simulink model "svpwm_model"  (R2024b)
settings: Solver=VariableStepAuto  StartTime=0.0  StopTime=10.0  RelTol=1e-3
undefined symbols (not defined in the file or in its folder): Ld, Lq, phi, pn
libraries: spsUniversalBridgeLib x1, spsPermanentMagnetSynchronousMachineLib x1, simulink x1, spsDCVoltageSourceLib x1, spsabctodq0Lib x1, spspowerguiLib x1

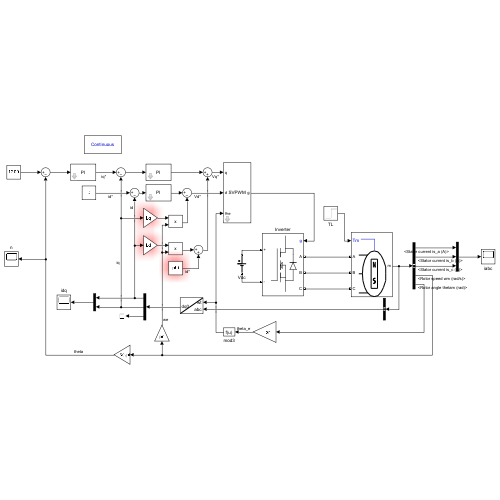
[thumbnail: Simulink's stored preview of the top-level diagram]
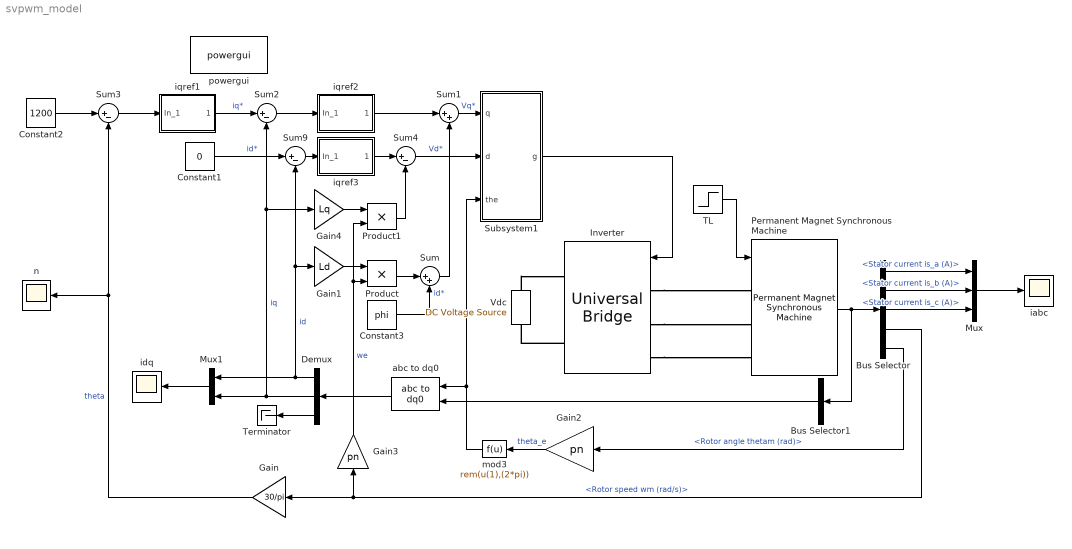
== system svpwm_model ==
  Bus Selector : BusSelector  OutputSignals=Stator current is_a (A),Stator current is_b (A),Stator current is_c (A),Rotor speed wm (rad/s),Rotor angle thetam (rad)
  Bus Selector1 : BusSelector  OutputSignals=Stator current is_a (A),Stator current is_b (A),Stator current is_c (A)  OutputAsBus=on
  Constant1 : Constant  Value=0
  Constant2 : Constant  Value=1200
  Constant3 : Constant  Value=phi
  Demux : Demux  Outputs=3
  Gain : Gain  Gain=30/pi
  Gain1 : Gain  Gain=Ld
  Gain2 : Gain  Gain=pn
  Gain3 : Gain  Gain=pn
  Gain4 : Gain  Gain=Lq
  Inverter : spsUniversalBridgeLib/Universal Bridge  Arms=3  SnubberResistance=1e5  SnubberCapacitance=inf  Device=MOSFET / Diodes  Ron=1e-3  Lon=0  ForwardVoltages="[  0  0  ]"  ForwardVoltage=0  GTOparameters=[ 10e-6 , 20e-6 ]  IGBTparameters=[ 1e-6 , 2e-6 ]  Measurements=None  Measurements_2=None  converterType=Rectifier
  Mux : Mux  Inputs=3
  Mux1 : Mux  Inputs=2
  Permanent Magnet Synchronous Machine : spsPermanentMagnetSynchronousMachineLib/Permanent Magnet Synchronous Machine  NbPhases=3  FluxDistribution=Sinusoidal  RotorType=Salient-pole  MechanicalLoad=Torque Tm  PresetModel="01:  0.8 Nm 300 Vdc 3000 RPM - 0.8 Nm"  ShowDetailedParameters=on  MeasurementBus=off  Resistance=18.7  Inductance=8.5e-3  dqInductances=[0.02547 0.02816]  La=0.000395  MachineConstant=Flux linkage established by magnets (V.s)  Flux=0.1716  VoltageCst=62.2496  TorqueCst=0.5148  Flat=120  Mechanical=[2.26e-05 1.349e-05 2 0]  PolePairs=2  InitialConditions=[0,0, 0,0]  InitialConditions5ph=[0 0 0 0 0 0]  RefAngle=Aligned with phase A axis (original Park)  IterativeDiscreteModel=Trapezoidal non iterative  TsBlock=-1  TsPowergui=0
  Product : Product
  Product1 : Product
  Subsystem1 : Subsystem  mask{Vdc=311}
  Sum : Sum  Inputs=|++
  Sum1 : Sum  Inputs=|++
  Sum{2..4,9} (4 alike) : Sum  Inputs=|+-
  TL : Step  Time=2  After=0.5  SampleTime=0
  Terminator : Terminator
  Vdc : spsDCVoltageSourceLib/DC Voltage Source  Amplitude=311  Measurements=None
  abc to dq0 : spsabctodq0Lib/abc to dq0  Alignment=Aligned with phase A axis
  iabc : Scope
  idq : Scope
  iqref1 : Subsystem  mask(PI Controller){I=20, P=0.15, sat=[-1, 1]}
      mask prompts: I "Integral"; P "Proportional:"; sat "Minimum and maximum outputs:"
      mask init:
      | min=sat(1);max=sat(2);
  iqref2 : Subsystem  mask(PI Controller){I=255, P=105, sat=[-311/2, 311/2]}
      mask prompts: I "Integral"; P "Proportional:"; sat "Minimum and maximum outputs:"
      mask init:
      | min=sat(1);max=sat(2);
  iqref3 : Subsystem  mask(PI Controller){I=255, P=105, sat=[-311/2,311/2]}
      mask prompts: I "Integral"; P "Proportional:"; sat "Minimum and maximum outputs:"
      mask init:
      | min=sat(1);max=sat(2);
  mod3 : Fcn  Expr=rem(u(1),(2*pi))
  n : Scope
  powergui : spspowerguiLib/powergui  Priority=1  SimulationMode=Continuous  SampleTime=10e-6  frequency=60  Iterations=50  frequencyindice=0  Pbase=100e6  ErrMax=1e-4  UnitsV=kV  UnitsW=MW  buscounter=0  FunctionMessages=off  echomessages=off  EnableUseOfTLC=off  CurrentSourceSwitches=off  DisableSnubberDevices=off  DisableRonSwitches=off  DisableVfSwitches=off  DisplayEquations=off  AutomaticDiscreteSolvers=off  SolverType=Tustin/Backward Euler (TBE)  Interpol=off  ExternalGateDelay=off  methode=off  Ts=100  x0status=blocks  SPID=on  SwTol=0  HookPort=off  NonlinearTolerance=1e-4  nMaxIteration=100  ContinueOnMaxIteration=off  RestoreLinks=warning  ResistiveCurrentMeasurement=off  Frange=[0:2:500]  Ylog=off  Xlog=on  ShowGrid=off  save=off  variable=ZData  structure=0  ZoomFFT=off  StartTime=0.0  cycles=1  DisplayStyle=1  fundamental=60  FreqAxis=off  MaxFrequency=1000  frequencyindicesteady=1  RmsSteady=1  display=off
  wires:
  Sum3/1 -> iqref1/1(In_1)
  Bus Selector/1 -> Mux/1  "<Stator current is_a (A)>"
  Mux/1 -> iabc/1
  abc to dq0/1 -> Demux/1
  Constant1/1 -> Sum9/1  "id*"
  Bus Selector/2 -> Mux/2  "<Stator current is_b (A)>"
  Gain/1 -> Sum3/2, n/1  "theta"
  iqref1/1(Out_1) -> Sum2/1  "iq*"
  mod3/1 -> Subsystem1/3(the), abc to dq0/2
  Bus Selector/4 -> Gain3/1, Gain/1  "<Rotor speed wm (rad/s)>"
  Demux/2 -> Sum2/2, Gain4/1, Mux1/2  "iq"
  Demux/3 -> Terminator/1
  Mux1/1 -> idq/1
  Subsystem1/1(g) -> Inverter/1
  Bus Selector/5 -> Gain2/1  "<Rotor angle thetam (rad)>"
  Sum9/1 -> iqref3/1(In_1)
  Sum2/1 -> iqref2/1(In_1)
  Bus Selector/3 -> Mux/3  "<Stator current is_c (A)>"
  Gain2/1 -> mod3/1  "theta_e"
  Bus Selector1/1 -> abc to dq0/1
  Constant2/1 -> Sum3/1
  TL/1 -> Permanent Magnet Synchronous Machine/1
  Permanent Magnet Synchronous Machine/1 -> Bus Selector1/1, Bus Selector/1
  Demux/1 -> Sum9/2, Gain1/1, Mux1/1  "id"
  iqref2/1(Out_1) -> Sum1/1
  Sum1/1 -> Subsystem1/1(q)  "Vq*"
  Gain3/1 -> Product1/2, Product/2  "we"
  Gain1/1 -> Product/1
  Product/1 -> Sum/1
  Constant3/1 -> Sum/2  "id*"
  Sum/1 -> Sum1/2
  iqref3/1(Out_1) -> Sum4/1
  Gain4/1 -> Product1/1
  Product1/1 -> Sum4/2
  Sum4/1 -> Subsystem1/2(d)  "Vd*"
  connections:
  Inverter/LConn2 -- Permanent Magnet Synchronous Machine/LConn2
  Inverter/LConn1 -- Permanent Magnet Synchronous Machine/LConn1
  Vdc/RConn1 -- Inverter/RConn1
  Inverter/LConn3 -- Permanent Magnet Synchronous Machine/LConn3
  Inverter/RConn2 -- Vdc/LConn1

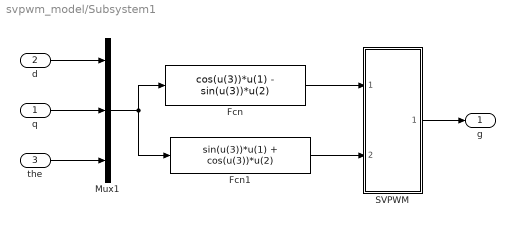
== system svpwm_model/Subsystem1 ==
  q : Inport
  d : Inport  Port=2
  the : Inport  Port=3
  Fcn : Fcn  Expr=cos(u(3))*u(1) - sin(u(3))*u(2)
  Fcn1 : Fcn  Expr=sin(u(3))*u(1) + cos(u(3))*u(2)
  Mux1 : Mux  Inputs=3
  SVPWM : Subsystem  Tag=SVPWM  mask{F=10, Vdc=311}
      mask prompts: F "Chopping　Frequency(KHz)"; Vdc "DC Voltage(V)"
  g : Outport
  wires:
  q/1 -> Mux1/2
  Fcn/1 -> SVPWM/1(Ualfa)
  d/1 -> Mux1/1
  Fcn1/1 -> SVPWM/2(Ubeta)
  SVPWM/1(pulse) -> g/1
  Mux1/1 -> Fcn/1, Fcn1/1
  the/1 -> Mux1/3

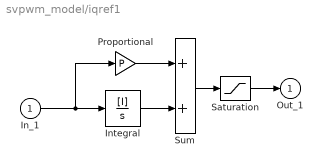
== system svpwm_model/iqref1 ==
  In_1 : Inport
  Integral : TransferFcn  Numerator=[I]  Denominator=[1 0]
  Proportional : Gain  Gain=P  SaturateOnIntegerOverflow=on  OutDataTypeStr=Inherit: Same as input  ParamDataTypeStr=Inherit: Same as input
  Saturation : Saturate  UpperLimit=max  LowerLimit=min
  Sum : Sum  InputSameDT=on  SaturateOnIntegerOverflow=on  OutDataTypeStr=Inherit: Same as first input
  Out_1 : Outport  InitialOutput=0  VectorParamsAs1DForOutWhenUnconnected=off
  wires:
  Saturation/1 -> Out_1/1
  Sum/1 -> Saturation/1
  Proportional/1 -> Sum/1
  In_1/1 -> Proportional/1, Integral/1
  Integral/1 -> Sum/2

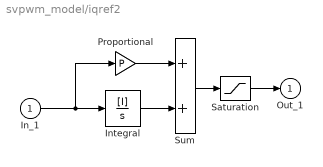
== system svpwm_model/iqref2 ==
  In_1 : Inport
  Integral : TransferFcn  Numerator=[I]  Denominator=[1 0]
  Proportional : Gain  Gain=P  SaturateOnIntegerOverflow=on  OutDataTypeStr=Inherit: Same as input  ParamDataTypeStr=Inherit: Same as input
  Saturation : Saturate  UpperLimit=max  LowerLimit=min
  Sum : Sum  InputSameDT=on  SaturateOnIntegerOverflow=on  OutDataTypeStr=Inherit: Same as first input
  Out_1 : Outport  InitialOutput=0  VectorParamsAs1DForOutWhenUnconnected=off
  wires:
  Saturation/1 -> Out_1/1
  Sum/1 -> Saturation/1
  Proportional/1 -> Sum/1
  In_1/1 -> Proportional/1, Integral/1
  Integral/1 -> Sum/2

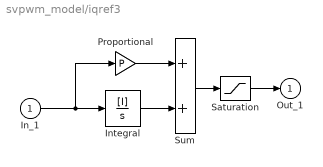
== system svpwm_model/iqref3 ==
  In_1 : Inport
  Integral : TransferFcn  Numerator=[I]  Denominator=[1 0]
  Proportional : Gain  Gain=P  SaturateOnIntegerOverflow=on  OutDataTypeStr=Inherit: Same as input  ParamDataTypeStr=Inherit: Same as input
  Saturation : Saturate  UpperLimit=max  LowerLimit=min
  Sum : Sum  InputSameDT=on  SaturateOnIntegerOverflow=on  OutDataTypeStr=Inherit: Same as first input
  Out_1 : Outport  InitialOutput=0  VectorParamsAs1DForOutWhenUnconnected=off
  wires:
  Saturation/1 -> Out_1/1
  Sum/1 -> Saturation/1
  Proportional/1 -> Sum/1
  In_1/1 -> Proportional/1, Integral/1
  Integral/1 -> Sum/2

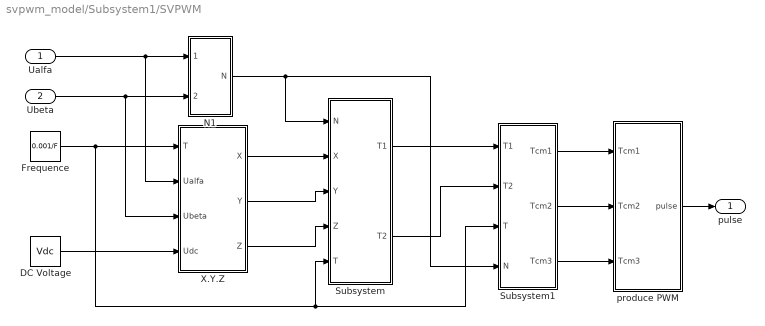
== system svpwm_model/Subsystem1/SVPWM ==
  Ualfa : Inport
  Ubeta : Inport  Port=2
  DC Voltage : Constant  Value=Vdc
  Frequence : Constant  Value=0.001/F
  N1 : Subsystem
  Subsystem : Subsystem
  Subsystem1 : Subsystem
  X.Y.Z : Subsystem
  produce PWM : Subsystem
  pulse : Outport
  wires:
  Ubeta/1 -> X.Y.Z/3(Ubeta), N1/2(Ubeta)
  Subsystem/2(T2) -> Subsystem1/2(T2)
  Subsystem/1(T1) -> Subsystem1/1(T1)
  Ualfa/1 -> N1/1(Ualfa), X.Y.Z/2(Ualfa)
  Subsystem1/3(Tcm3) -> produce PWM/3(Tcm3)
  Subsystem1/2(Tcm2) -> produce PWM/2(Tcm2)
  Subsystem1/1(Tcm1) -> produce PWM/1(Tcm1)
  X.Y.Z/3(Z) -> Subsystem/4(Z)
  X.Y.Z/2(Y) -> Subsystem/3(Y)
  X.Y.Z/1(X) -> Subsystem/2(X)
  N1/1(N) -> Subsystem1/4(N), Subsystem/1(N)
  DC Voltage/1 -> X.Y.Z/4(Udc)
  Frequence/1 -> Subsystem/5(T), Subsystem1/3(T), X.Y.Z/1(T)
  produce PWM/1(pulse) -> pulse/1

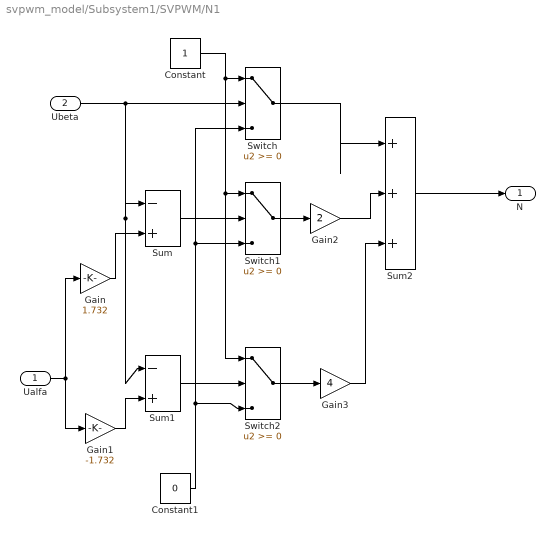
== system svpwm_model/Subsystem1/SVPWM/N1 ==
  Ualfa : Inport
  Ubeta : Inport  Port=2
  Constant : Constant
  Constant1 : Constant  Value=0
  Gain : Gain  Gain=1.732
  Gain1 : Gain  Gain=-1.732
  Gain2 : Gain  Gain=2
  Gain3 : Gain  Gain=4
  Sum : Sum  Inputs=|-+
  Sum1 : Sum  Inputs=|-+
  Sum2 : Sum  Inputs=|+++
  Switch : Switch  SaturateOnIntegerOverflow=off  InputSameDT=off
  Switch1 : Switch  SaturateOnIntegerOverflow=off  InputSameDT=off
  Switch2 : Switch  SaturateOnIntegerOverflow=off  InputSameDT=off
  N : Outport
  wires:
  Sum2/1 -> N/1
  Gain3/1 -> Sum2/3
  Switch/1 -> Sum2/1
  Gain2/1 -> Sum2/2
  Switch2/1 -> Gain3/1
  Switch1/1 -> Gain2/1
  Constant1/1 -> Switch2/3, Switch1/3, Switch/3
  Gain1/1 -> Sum1/2
  Sum1/1 -> Switch2/2
  Sum/1 -> Switch1/2
  Gain/1 -> Sum/2
  Ualfa/1 -> Gain/1, Gain1/1
  Constant/1 -> Switch1/1, Switch2/1, Switch/1
  Ubeta/1 -> Sum1/1, Sum/1, Switch/2

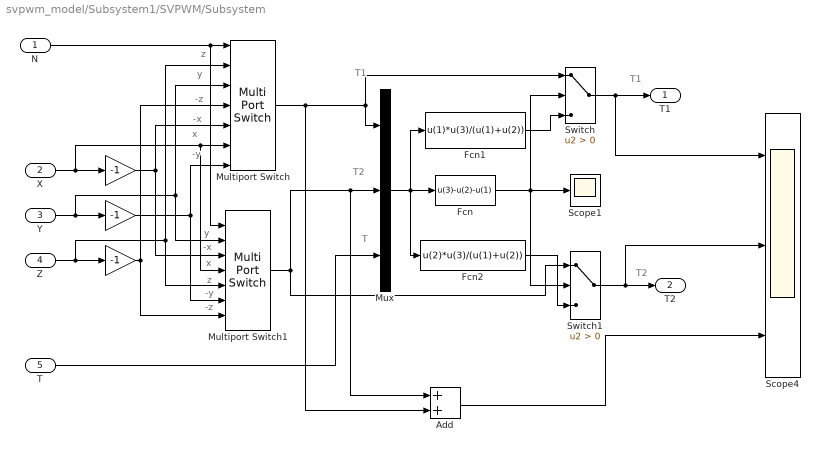
== system svpwm_model/Subsystem1/SVPWM/Subsystem ==
  note: T2
  note: T1
  note: T
  note: T2
  note: T1
  note: -z
  note: -y
  note: z
  note: x
  note: -x
  note: y
  note: -y
  note: x
  note: -x
  note: -z
  note: y
  note: z
  N : Inport
  X : Inport  Port=2
  Y : Inport  Port=3
  Z : Inport  Port=4
  T : Inport  Port=5
  " " : Gain  Gain=-1
  "  " : Gain  Gain=-1
  "    " : Gain  Gain=-1
  Add : Sum
  Fcn : Fcn  Expr=u(3)-u(2)-u(1)
  Fcn1 : Fcn  Expr=u(1)*u(3)/(u(1)+u(2))
  Fcn2 : Fcn  Expr=u(2)*u(3)/(u(1)+u(2))
  Multiport Switch : MultiPortSwitch  Inputs=6  DiagnosticForDefault=None  SaturateOnIntegerOverflow=off  InputSameDT=off
  Multiport Switch1 : MultiPortSwitch  Inputs=6  DiagnosticForDefault=None  SaturateOnIntegerOverflow=off  InputSameDT=off
  Mux : Mux  Inputs=3
  Scope1 : Scope
  Scope4 : Scope  NumInputPorts=3
  Switch : Switch  Criteria=u2 > Threshold  SaturateOnIntegerOverflow=off  InputSameDT=off
  Switch1 : Switch  Criteria=u2 > Threshold  SaturateOnIntegerOverflow=off  InputSameDT=off
  T1 : Outport
  T2 : Outport  Port=2
  wires:
  Add/1 -> Scope4/3
  Switch1/1 -> Scope4/2, T2/1
  Switch/1 -> Scope4/1, T1/1
  Fcn2/1 -> Switch1/3
  Fcn1/1 -> Switch/3
  Mux/1 -> Fcn2/1, Fcn1/1, Fcn/1
  T/1 -> Mux/3
  Multiport Switch/1 -> Add/2, Switch/1, Mux/1
  " "/1 -> Multiport Switch1/3, Multiport Switch/5
  "  "/1 -> Multiport Switch1/6, Multiport Switch/7
  "    "/1 -> Multiport Switch/4, Multiport Switch1/7
  Z/1 -> "    "/1, Multiport Switch/2, Multiport Switch1/5
  Y/1 -> "  "/1, Multiport Switch/3, Multiport Switch1/2
  X/1 -> " "/1, Multiport Switch/6, Multiport Switch1/4
  N/1 -> Multiport Switch/1, Multiport Switch1/1
  Fcn/1 -> Scope1/1, Switch1/2, Switch/2
  Multiport Switch1/1 -> Add/1, Mux/2, Switch1/1

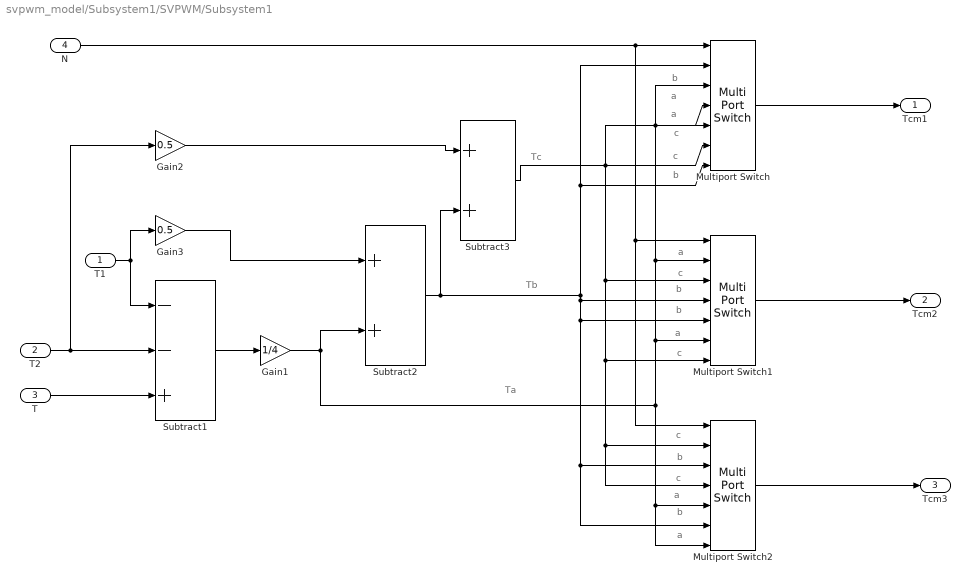
== system svpwm_model/Subsystem1/SVPWM/Subsystem1 ==
  note: a
  note: b
  note: a
  note: c
  note: b
  note: c
  note: c
  note: a
  note: b
  note: b
  note: c
  note: a
  note: b
  note: c
  note: c
  note: a
  note: a
  note: b
  note: Tc
  note: Tb
  note: Ta
  T1 : Inport
  T2 : Inport  Port=2
  T : Inport  Port=3
  N : Inport  Port=4
  Gain1 : Gain  Gain=1/4
  Gain2 : Gain  Gain=0.5
  Gain3 : Gain  Gain=0.5
  Multiport Switch : MultiPortSwitch  Inputs=6  DiagnosticForDefault=None  SaturateOnIntegerOverflow=off  InputSameDT=off
  Multiport Switch1 : MultiPortSwitch  Inputs=6  DiagnosticForDefault=None  SaturateOnIntegerOverflow=off  InputSameDT=off
  Multiport Switch2 : MultiPortSwitch  Inputs=6  DiagnosticForDefault=None  SaturateOnIntegerOverflow=off  InputSameDT=off
  Subtract1 : Sum  Inputs=--+
  Subtract2 : Sum
  Subtract3 : Sum
  Tcm1 : Outport
  Tcm2 : Outport  Port=2
  Tcm3 : Outport  Port=3
  wires:
  Subtract3/1 -> Multiport Switch2/4, Multiport Switch2/2, Multiport Switch1/7, Multiport Switch1/3, Multiport Switch/6, Multiport Switch/5
  N/1 -> Multiport Switch1/1, Multiport Switch2/1, Multiport Switch/1
  Gain2/1 -> Subtract3/1
  Subtract2/1 -> Multiport Switch2/6, Multiport Switch2/3, Multiport Switch1/5, Multiport Switch1/4, Multiport Switch/7, Multiport Switch/2, Subtract3/2
  Gain1/1 -> Subtract2/2, Multiport Switch1/6, Multiport Switch1/2, Multiport Switch/4, Multiport Switch/3, Multiport Switch2/7, Multiport Switch2/5
  Subtract1/1 -> Gain1/1
  Gain3/1 -> Subtract2/1
  T1/1 -> Subtract1/1, Gain3/1
  T/1 -> Subtract1/3
  T2/1 -> Subtract1/2, Gain2/1
  Multiport Switch/1 -> Tcm1/1
  Multiport Switch1/1 -> Tcm2/1
  Multiport Switch2/1 -> Tcm3/1

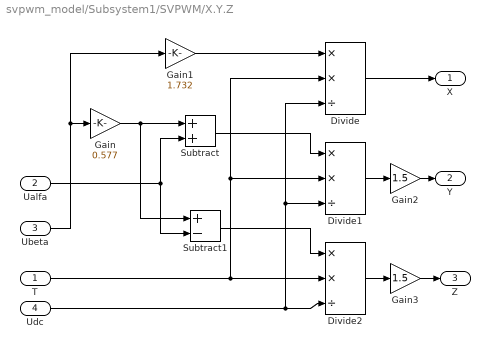
== system svpwm_model/Subsystem1/SVPWM/X.Y.Z ==
  T : Inport
  Ualfa : Inport  Port=2
  Ubeta : Inport  Port=3
  Udc : Inport  Port=4
  Divide : Product  Inputs=**/
  Divide1 : Product  Inputs=**/
  Divide2 : Product  Inputs=**/
  Gain : Gain  Gain=0.577
  Gain1 : Gain  Gain=1.732
  Gain2 : Gain  Gain=1.5
  Gain3 : Gain  Gain=1.5
  Subtract : Sum
  Subtract1 : Sum  Inputs=+-
  X : Outport
  Y : Outport  Port=2
  Z : Outport  Port=3
  wires:
  Ubeta/1 -> Gain/1, Gain1/1
  Gain3/1 -> Z/1
  Gain2/1 -> Y/1
  Divide2/1 -> Gain3/1
  Divide1/1 -> Gain2/1
  Divide/1 -> X/1
  Subtract1/1 -> Divide2/1
  Subtract/1 -> Divide1/1
  Ualfa/1 -> Subtract/2, Subtract1/2
  Udc/1 -> Divide/3, Divide1/3, Divide2/3
  T/1 -> Divide/2, Divide1/2, Divide2/2
  Gain1/1 -> Divide/1
  Gain/1 -> Subtract1/1, Subtract/1

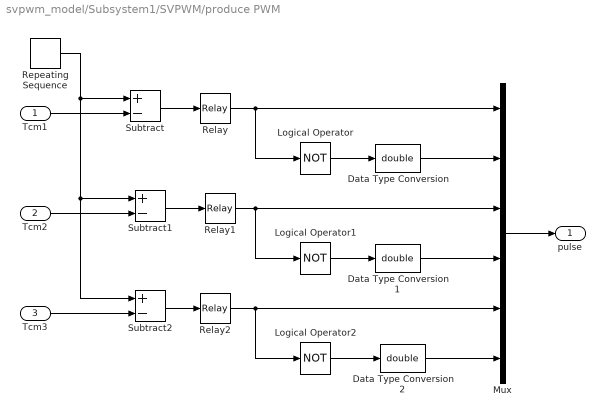
== system svpwm_model/Subsystem1/SVPWM/produce PWM ==
  Tcm1 : Inport
  Tcm2 : Inport  Port=2
  Tcm3 : Inport  Port=3
  Data Type Conversion : DataTypeConversion  OutDataTypeStr=double  SaturateOnIntegerOverflow=off  RndMeth=Floor
  Data Type Conversion1 : DataTypeConversion  OutDataTypeStr=double  SaturateOnIntegerOverflow=off  RndMeth=Floor
  Data Type Conversion2 : DataTypeConversion  OutDataTypeStr=double  SaturateOnIntegerOverflow=off  RndMeth=Floor
  Logical Operator : Logic  Operator=NOT  AllPortsSameDT=off
  Logical Operator1 : Logic  Operator=NOT  AllPortsSameDT=off
  Logical Operator2 : Logic  Operator=NOT  AllPortsSameDT=off
  Mux : Mux  Inputs=6
  Relay : Relay
  Relay1 : Relay
  Relay2 : Relay
  Repeating Sequence : simulink/Sources/Repeating Sequence  rep_seq_t=[0 0.001/F 0.002/F]  rep_seq_y=[0 0.001/F 0]
  Subtract : Sum  Inputs=+-
  Subtract1 : Sum  Inputs=+-
  Subtract2 : Sum  Inputs=+-
  pulse : Outport
  wires:
  Data Type Conversion2/1 -> Mux/6
  Data Type Conversion1/1 -> Mux/4
  Data Type Conversion/1 -> Mux/2
  Mux/1 -> pulse/1
  Relay2/1 -> Mux/5, Logical Operator2/1
  Relay1/1 -> Mux/3, Logical Operator1/1
  Relay/1 -> Mux/1, Logical Operator/1
  Logical Operator/1 -> Data Type Conversion/1
  Logical Operator2/1 -> Data Type Conversion2/1
  Logical Operator1/1 -> Data Type Conversion1/1
  Tcm3/1 -> Subtract2/2
  Tcm2/1 -> Subtract1/2
  Tcm1/1 -> Subtract/2
  Repeating Sequence/1 -> Subtract1/1, Subtract2/1, Subtract/1
  Subtract2/1 -> Relay2/1
  Subtract1/1 -> Relay1/1
  Subtract/1 -> Relay/1
